simulink model "Flap"  (R2024b)
settings: Solver=ode45  StartTime=0  StopTime=400  FixedStep=0.1  MaxStep=0.1  EnableMultiTasking=on
values from neighbouring files (symbols this model uses):
  Ki = -2*pi/5*imag(1/H(1)')    [BranchAndBound.m]    (also in Optimization.m; RectangularOptimization.m; RoundingPI.m; wecSimInputFile.m = -100000)
  Kp = real(1/H(1)')    [BranchAndBound.m]    (also in Optimization.m; RectangularOptimization.m; RoundingPI.m; wecSimInputFile.m = 500000)
  params = struct    [BranchAndBound.m]    (also in Optimization.m; Parameters.m = struct(); RectangularOptimization.m; RoundingPI.m)
  PTO = 'Continuous PI'    [wecSimInputFile.m]
  valveTransferFunction = tf(4/valveSettlingTime,[1 4/valveSettlingTime])    [Parameters.m]
undefined symbols (not defined in the file or in its folder): body, constraint, geometry, hydroData, pressure, pto, ptoSim
libraries: WECSim_Lib_Body_Elements x2, WECSim_Lib_Constraints x1, WECSim_Lib_Frames x1, simulink x1, WECSim_Lib_PTOSim x1, WECSim_Lib_PTOs x1
(part 2 of 2)

== system Flap/PTO/Active Valving/capValves/Subsystem1 ==
  Pin : Inport
  Pout : Inport  Port=2
  valveCommand : Inport  Port=3
  MATLAB Function : MATLAB Function  TreatAsAtomicUnit=on
  flow : Outport
  loss : Outport  Port=2
  wires:
  MATLAB Function/1(flow) -> flow/1
  valveCommand/1 -> MATLAB Function/3(valveCommand)
  Pout/1 -> MATLAB Function/2(Pout)
  Pin/1 -> MATLAB Function/1(Pin)
  MATLAB Function/2(loss) -> loss/1

== system Flap/PTO/Active Valving/capValves/Subsystem2 ==
  Pin : Inport
  Pout : Inport  Port=2
  valveCommand : Inport  Port=3
  MATLAB Function : MATLAB Function  TreatAsAtomicUnit=on
  flow : Outport
  loss : Outport  Port=2
  wires:
  MATLAB Function/1(flow) -> flow/1
  valveCommand/1 -> MATLAB Function/3(valveCommand)
  Pout/1 -> MATLAB Function/2(Pout)
  Pin/1 -> MATLAB Function/1(Pin)
  MATLAB Function/2(loss) -> loss/1

== system Flap/PTO/Active Valving/rodValves/Subsystem ==
  Pin : Inport
  Pout : Inport  Port=2
  valveCommand : Inport  Port=3
  MATLAB Function : MATLAB Function  TreatAsAtomicUnit=on
  flow : Outport
  loss : Outport  Port=2
  wires:
  MATLAB Function/1(flow) -> flow/1
  valveCommand/1 -> MATLAB Function/3(valveCommand)
  Pout/1 -> MATLAB Function/2(Pout)
  Pin/1 -> MATLAB Function/1(Pin)
  MATLAB Function/2(loss) -> loss/1

== system Flap/PTO/Active Valving/rodValves/Subsystem1 ==
  Pin : Inport
  Pout : Inport  Port=2
  valveCommand : Inport  Port=3
  MATLAB Function : MATLAB Function  TreatAsAtomicUnit=on
  flow : Outport
  loss : Outport  Port=2
  wires:
  MATLAB Function/1(flow) -> flow/1
  valveCommand/1 -> MATLAB Function/3(valveCommand)
  Pout/1 -> MATLAB Function/2(Pout)
  Pin/1 -> MATLAB Function/1(Pin)
  MATLAB Function/2(loss) -> loss/1

== system Flap/PTO/Active Valving/rodValves/Subsystem2 ==
  Pin : Inport
  Pout : Inport  Port=2
  valveCommand : Inport  Port=3
  MATLAB Function : MATLAB Function  TreatAsAtomicUnit=on
  flow : Outport
  loss : Outport  Port=2
  wires:
  MATLAB Function/1(flow) -> flow/1
  valveCommand/1 -> MATLAB Function/3(valveCommand)
  Pout/1 -> MATLAB Function/2(Pout)
  Pin/1 -> MATLAB Function/1(Pin)
  MATLAB Function/2(loss) -> loss/1

== system Flap/PTO/EHA/Subsystem/CapPressureDynamics ==
  position : Inport
  velocity : Inport  Port=2
  flow : Inport  Port=3
  Gain : Gain  Gain=params.capArea
  Integrator : Integrator  LimitOutput=on  UpperSaturationLimit=30e6  LowerSaturationLimit=0
  MATLAB Function : MATLAB Function  TreatAsAtomicUnit=on
  Scope : Scope  NumInputPorts=3
  Subtract : Sum  Inputs=+-
  capPressure : Outport
  wires:
  MATLAB Function/1(pressure_dot) -> Integrator/1
  Integrator/1 -> capPressure/1  "capPressure"
  flow/1 -> Scope/2, Subtract/1, MATLAB Function/3(flow)
  velocity/1 -> Gain/1, MATLAB Function/2(velocity)
  position/1 -> MATLAB Function/1(position)
  Gain/1 -> Subtract/2, Scope/1  "capdV"
  Subtract/1 -> Scope/3  "capQ_dV"

== system Flap/PTO/EHA/Subsystem/HECM ==
  note: dP = capPressure - rodPressure
  displacementCommand : Inport
  rodPressure : Inport  Port=2
  capPressure : Inport  Port=3
  Gain : Gain  Gain=-1
  MATLAB Function : MATLAB Function  TreatAsAtomicUnit=on
  Subtract : Sum  Inputs=+-
  Terminator : Terminator
  Terminator1 : Terminator
  To Workspace : ToWorkspace  VariableName=electricPower  SampleTime=-1
  capFlow : Outport
  rodFlow : Outport  Port=2
  wires:
  Subtract/1 -> MATLAB Function/2(dp)  "dP_actual"
  MATLAB Function/1(Loss) -> Terminator/1  "Loss"
  rodPressure/1 -> Subtract/2
  displacementCommand/1 -> MATLAB Function/1(x)
  MATLAB Function/2(Q) -> rodFlow/1, Gain/1  "rodFlow"
  capPressure/1 -> Subtract/1
  Gain/1 -> capFlow/1  "capFlow"
  MATLAB Function/3(elecPower) -> To Workspace/1, Terminator1/1  "electricPower"

== system Flap/PTO/EHA/Subsystem/RodPressureDynamics ==
  velocity : Inport
  position : Inport  Port=2
  flow : Inport  Port=3
  Integrator : Integrator  LimitOutput=on  UpperSaturationLimit=30e6  LowerSaturationLimit=0
  MATLAB Function : MATLAB Function  TreatAsAtomicUnit=on
  rodPressure : Outport
  wires:
  position/1 -> MATLAB Function/1(position)
  velocity/1 -> MATLAB Function/2(velocity)
  flow/1 -> MATLAB Function/3(flow)
  Integrator/1 -> rodPressure/1  "rodPressure"
  MATLAB Function/1(pressure_dot) -> Integrator/1  "rodPressureDot"

== system Flap/PTO/HHEA/Subsystem/CapPressureDynamics ==
  position : Inport
  velocity : Inport  Port=2
  flow : Inport  Port=3
  Integrator : Integrator
  MATLAB Function : MATLAB Function  TreatAsAtomicUnit=on
  capPressure : Outport
  wires:
  MATLAB Function/1(pressure_dot) -> Integrator/1
  Integrator/1 -> capPressure/1  "capPressure"
  flow/1 -> MATLAB Function/3(flow)
  velocity/1 -> MATLAB Function/2(velocity)
  position/1 -> MATLAB Function/1(position)

== system Flap/PTO/HHEA/Subsystem/HECM ==
  note: dP = rodValvePressure - rodPressure
      | (+) positive dP and torque causes positive flow and speed, which causes increased pressure in the rod chamber
  flowIn : Inport
  speedCommand : Inport  Port=2
  rodPressure : Inport  Port=3
  Integrator : Integrator
  MATLAB Function : MATLAB Function  TreatAsAtomicUnit=on
  MATLAB Function1 : MATLAB Function  TreatAsAtomicUnit=on
  Scope : Scope  NumInputPorts=2
  Scope1 : Scope  NumInputPorts=2
  Subtract : Sum  Inputs=+-
  Terminator : Terminator
  flowOut : Outport
  rodValvePressure : Outport  Port=2
  wires:
  Subtract/1 -> Scope/1, MATLAB Function/2(dp)  "dP_actual"
  MATLAB Function/1(Loss) -> Terminator/1
  MATLAB Function/3(dp_ideal) -> Scope/2
  MATLAB Function/4(w_ideal) -> Scope1/2
  rodPressure/1 -> Subtract/2
  speedCommand/1 -> Scope1/1, MATLAB Function/1(w)
  MATLAB Function/2(Q) -> MATLAB Function1/2(Q_out), flowOut/1  "rodFlow"
  MATLAB Function1/1(Pdot) -> Integrator/1
  Integrator/1 -> Subtract/1, rodValvePressure/1  "rodValvePressure"
  flowIn/1 -> MATLAB Function1/1(Q_in)

== system Flap/PTO/HHEA/Subsystem/PressureRails ==
  note: flow into the rails
  capRailFlow : Inport
  rodRailFlow : Inport  Port=2
  Constant : Constant  Value=35e6
  Constant3 : Constant  Value=17.5e6
  Constant4 : Constant  Value=0
  Mux : Mux  Inputs=3
  Product : Product
  Sum : Sum  Inputs=|++
  Sum of Elements : Sum  Inputs=+
  To Workspace : ToWorkspace  VariableName=railPower  SampleTime=-1
  pressureRails : Outport
  wires:
  Sum/1 -> Product/1
  Product/1 -> Sum of Elements/1
  Sum of Elements/1 -> To Workspace/1
  rodRailFlow/1 -> Sum/2
  capRailFlow/1 -> Sum/1
  Constant3/1 -> Mux/2
  Constant4/1 -> Mux/1
  Constant/1 -> Mux/3
  Mux/1 -> Product/2, pressureRails/1

== system Flap/PTO/HHEA/Subsystem/RodPressureDynamics ==
  velocity : Inport
  position : Inport  Port=2
  flow : Inport  Port=3
  Gain : Gain  Gain=-params.rodArea
  Integrator : Integrator
  MATLAB Function : MATLAB Function  TreatAsAtomicUnit=on
  Scope : Scope  NumInputPorts=2
  Scope1 : Scope  NumInputPorts=2
  Scope2 : Scope
  Sum : Sum  Inputs=|++
  rodPressure : Outport
  wires:
  position/1 -> MATLAB Function/1(position)
  velocity/1 -> MATLAB Function/2(velocity), Gain/1
  flow/1 -> Sum/2, Scope1/2, MATLAB Function/3(flow)
  Integrator/1 -> Scope/2, rodPressure/1  "rodPressure"
  MATLAB Function/1(pressure_dot) -> Scope/1, Integrator/1  "rodPressureDot"
  Gain/1 -> Sum/1, Scope1/1
  Sum/1 -> Scope2/1

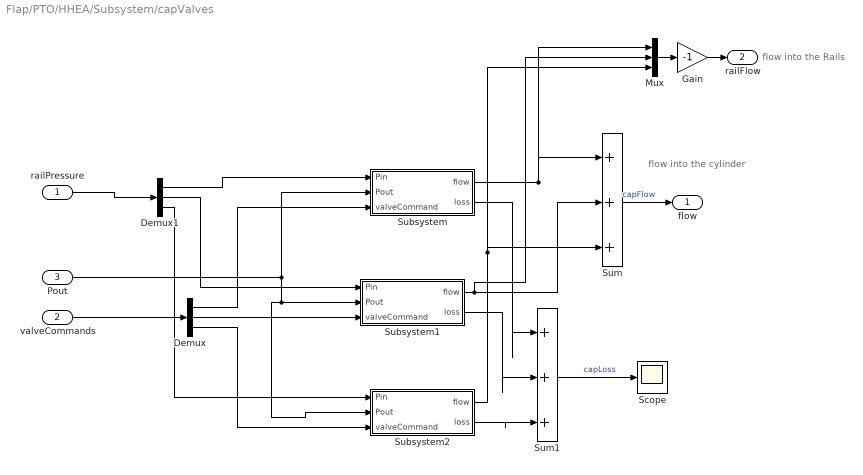
== system Flap/PTO/HHEA/Subsystem/capValves ==
  note: flow into the cylinder
  note: flow into the Rails
  railPressure : Inport
  valveCommands : Inport  Port=2
  Pout : Inport  Port=3
  Demux : Demux  Outputs=3
  Demux1 : Demux  Outputs=3
  Gain : Gain  Gain=-1
  Mux : Mux  Inputs=3
  Scope : Scope
  Subsystem : Subsystem
  Subsystem1 : Subsystem
  Subsystem2 : Subsystem
  Sum : Sum  Inputs=|+++
  Sum1 : Sum  Inputs=|+++
  flow : Outport
  railFlow : Outport  Port=2
  wires:
  Pout/1 -> Subsystem/2(Pout), Subsystem2/2(Pout), Subsystem1/2(Pout)
  valveCommands/1 -> Demux/1
  Demux/1 -> Subsystem/3(valveCommand)
  Demux/2 -> Subsystem1/3(valveCommand)
  Demux/3 -> Subsystem2/3(valveCommand)
  Sum/1 -> flow/1  "capFlow"
  Subsystem/2(loss) -> Sum1/1
  Subsystem1/2(loss) -> Sum1/2
  Subsystem2/2(loss) -> Sum1/3
  Sum1/1 -> Scope/1  "capLoss"
  railPressure/1 -> Demux1/1
  Demux1/1 -> Subsystem/1(Pin)
  Demux1/2 -> Subsystem1/1(Pin)
  Demux1/3 -> Subsystem2/1(Pin)
  Subsystem1/1(flow) -> Mux/2, Sum/2
  Mux/1 -> Gain/1
  Subsystem2/1(flow) -> Mux/3, Sum/3
  Subsystem/1(flow) -> Mux/1, Sum/1
  Gain/1 -> railFlow/1

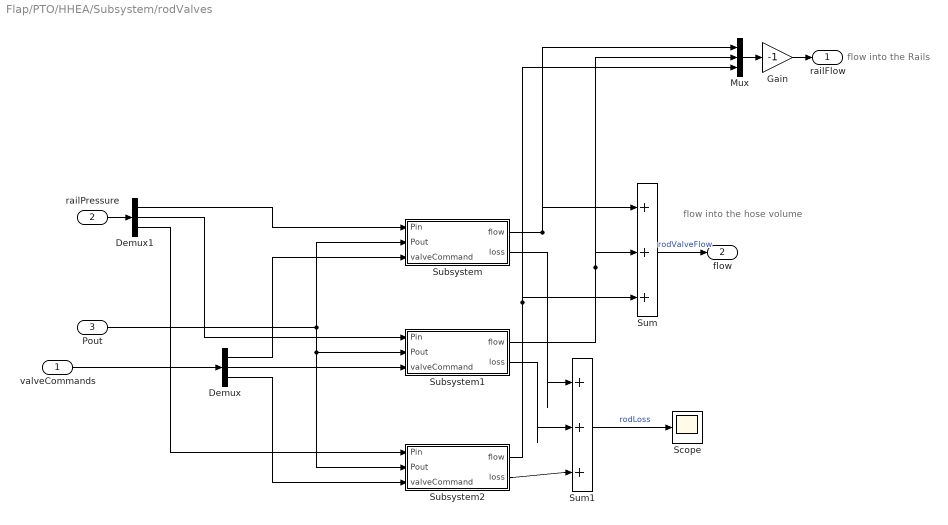
== system Flap/PTO/HHEA/Subsystem/rodValves ==
  note: flow into the hose volume
  note: flow into the Rails
  valveCommands : Inport
  railPressure : Inport  Port=2
  Pout : Inport  Port=3
  Demux : Demux  Outputs=3
  Demux1 : Demux  Outputs=3
  Gain : Gain  Gain=-1
  Mux : Mux  Inputs=3
  Scope : Scope
  Subsystem : Subsystem
  Subsystem1 : Subsystem
  Subsystem2 : Subsystem
  Sum : Sum  Inputs=|+++
  Sum1 : Sum  Inputs=|+++
  railFlow : Outport
  flow : Outport  Port=2
  wires:
  Pout/1 -> Subsystem/2(Pout), Subsystem2/2(Pout), Subsystem1/2(Pout)
  valveCommands/1 -> Demux/1
  Demux/1 -> Subsystem/3(valveCommand)
  Demux1/2 -> Subsystem1/1(Pin)
  Demux1/3 -> Subsystem2/1(Pin)
  Demux/2 -> Subsystem1/3(valveCommand)
  Demux/3 -> Subsystem2/3(valveCommand)
  Sum/1 -> flow/1  "rodValveFlow"
  Subsystem/2(loss) -> Sum1/1
  Subsystem1/2(loss) -> Sum1/2
  Subsystem2/2(loss) -> Sum1/3
  Sum1/1 -> Scope/1  "rodLoss"
  railPressure/1 -> Demux1/1
  Demux1/1 -> Subsystem/1(Pin)
  Subsystem1/1(flow) -> Mux/2, Sum/2
  Mux/1 -> Gain/1
  Subsystem2/1(flow) -> Mux/3, Sum/3
  Subsystem/1(flow) -> Mux/1, Sum/1
  Gain/1 -> railFlow/1

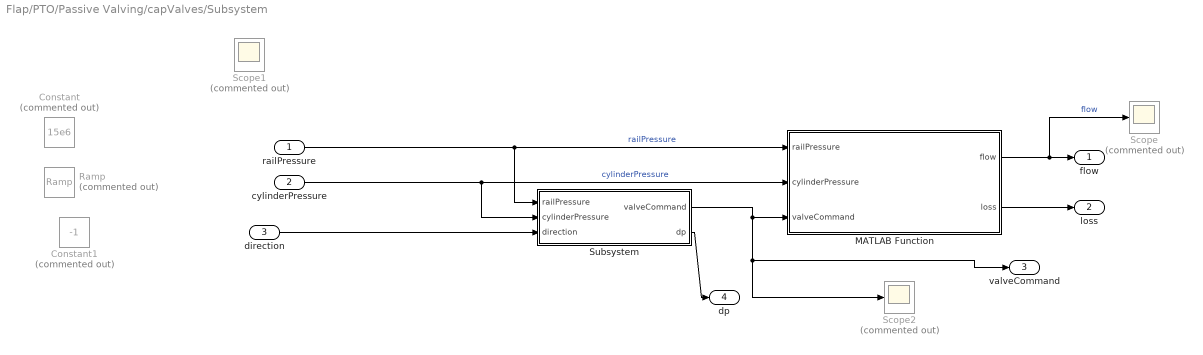
== system Flap/PTO/Passive Valving/capValves/Subsystem ==
  railPressure : Inport
  cylinderPressure : Inport  Port=2
  direction : Inport  Port=3
  Constant : Constant  Commented=on  Value=15e6
  Constant1 : Constant  Commented=on  Value=-1
  MATLAB Function : MATLAB Function  TreatAsAtomicUnit=on
  Ramp : simulink/Sources/Ramp  Commented=on  slope=-1e6  start=0  InitialOutput=20e6
  Scope : Scope  Commented=on
  Scope1 : Scope  Commented=on  NumInputPorts=2
  Scope2 : Scope  Commented=on
  Subsystem : Subsystem
  flow : Outport
  loss : Outport  Port=2
  valveCommand : Outport  Port=3
  dp : Outport  Port=4
  wires:
  railPressure/1 -> Subsystem/1(railPressure), MATLAB Function/1(railPressure)  "railPressure"
  Subsystem/1(valveCommand) -> valveCommand/1, Scope2/1, MATLAB Function/3(valveCommand)
  MATLAB Function/1(flow) -> Scope/1, flow/1  "flow"
  Subsystem/2(dp) -> dp/1
  MATLAB Function/2(loss) -> loss/1
  direction/1 -> Subsystem/3(direction)
  cylinderPressure/1 -> MATLAB Function/2(cylinderPressure), Subsystem/2(cylinderPressure)  "cylinderPressure"

== system Flap/PTO/HHEA/Subsystem/capValves/Subsystem ==
  Pin : Inport
  Pout : Inport  Port=2
  valveCommand : Inport  Port=3
  MATLAB Function : MATLAB Function  TreatAsAtomicUnit=on
  Transfer Fcn : TransferFcn  Numerator=valveTransferFunction.Numerator{1}  Denominator=valveTransferFunction.Denominator{1}
  flow : Outport
  loss : Outport  Port=2
  wires:
  MATLAB Function/1(flow) -> flow/1
  valveCommand/1 -> Transfer Fcn/1
  Pout/1 -> MATLAB Function/2(Pout)
  Pin/1 -> MATLAB Function/1(Pin)
  MATLAB Function/2(loss) -> loss/1
  Transfer Fcn/1 -> MATLAB Function/3(valveCommand)

== system Flap/PTO/HHEA/Subsystem/capValves/Subsystem1 ==
  Pin : Inport
  Pout : Inport  Port=2
  valveCommand : Inport  Port=3
  MATLAB Function : MATLAB Function  TreatAsAtomicUnit=on
  Transfer Fcn : TransferFcn  Numerator=valveTransferFunction.Numerator{1}  Denominator=valveTransferFunction.Denominator{1}
  flow : Outport
  loss : Outport  Port=2
  wires:
  MATLAB Function/1(flow) -> flow/1
  valveCommand/1 -> Transfer Fcn/1
  Pout/1 -> MATLAB Function/2(Pout)
  Pin/1 -> MATLAB Function/1(Pin)
  MATLAB Function/2(loss) -> loss/1
  Transfer Fcn/1 -> MATLAB Function/3(valveCommand)

== system Flap/PTO/HHEA/Subsystem/capValves/Subsystem2 ==
  Pin : Inport
  Pout : Inport  Port=2
  valveCommand : Inport  Port=3
  MATLAB Function : MATLAB Function  TreatAsAtomicUnit=on
  Transfer Fcn : TransferFcn  Numerator=valveTransferFunction.Numerator{1}  Denominator=valveTransferFunction.Denominator{1}
  flow : Outport
  loss : Outport  Port=2
  wires:
  MATLAB Function/1(flow) -> flow/1
  valveCommand/1 -> Transfer Fcn/1
  Pout/1 -> MATLAB Function/2(Pout)
  Pin/1 -> MATLAB Function/1(Pin)
  MATLAB Function/2(loss) -> loss/1
  Transfer Fcn/1 -> MATLAB Function/3(valveCommand)

== system Flap/PTO/HHEA/Subsystem/rodValves/Subsystem ==
  Pin : Inport
  Pout : Inport  Port=2
  valveCommand : Inport  Port=3
  MATLAB Function : MATLAB Function  TreatAsAtomicUnit=on
  Transfer Fcn : TransferFcn  Numerator=valveTransferFunction.Numerator{1}  Denominator=valveTransferFunction.Denominator{1}
  flow : Outport
  loss : Outport  Port=2
  wires:
  MATLAB Function/1(flow) -> flow/1
  valveCommand/1 -> Transfer Fcn/1
  Pout/1 -> MATLAB Function/2(Pout)
  Pin/1 -> MATLAB Function/1(Pin)
  MATLAB Function/2(loss) -> loss/1
  Transfer Fcn/1 -> MATLAB Function/3(valveCommand)

== system Flap/PTO/HHEA/Subsystem/rodValves/Subsystem1 ==
  Pin : Inport
  Pout : Inport  Port=2
  valveCommand : Inport  Port=3
  MATLAB Function : MATLAB Function  TreatAsAtomicUnit=on
  Transfer Fcn : TransferFcn  Numerator=valveTransferFunction.Numerator{1}  Denominator=valveTransferFunction.Denominator{1}
  flow : Outport
  loss : Outport  Port=2
  wires:
  MATLAB Function/1(flow) -> flow/1
  valveCommand/1 -> Transfer Fcn/1
  Pout/1 -> MATLAB Function/2(Pout)
  Pin/1 -> MATLAB Function/1(Pin)
  MATLAB Function/2(loss) -> loss/1
  Transfer Fcn/1 -> MATLAB Function/3(valveCommand)

== system Flap/PTO/HHEA/Subsystem/rodValves/Subsystem2 ==
  Pin : Inport
  Pout : Inport  Port=2
  valveCommand : Inport  Port=3
  MATLAB Function : MATLAB Function  TreatAsAtomicUnit=on
  Transfer Fcn : TransferFcn  Numerator=valveTransferFunction.Numerator{1}  Denominator=valveTransferFunction.Denominator{1}
  flow : Outport
  loss : Outport  Port=2
  wires:
  MATLAB Function/1(flow) -> flow/1
  valveCommand/1 -> Transfer Fcn/1
  Pout/1 -> MATLAB Function/2(Pout)
  Pin/1 -> MATLAB Function/1(Pin)
  MATLAB Function/2(loss) -> loss/1
  Transfer Fcn/1 -> MATLAB Function/3(valveCommand)

== system Flap/PTO/Passive Valving/capValves/Subsystem/Subsystem ==
  note: dp = inlet - outlet
      | Positive dp tends to open the valve and cause flow from the inlet to the outlet
  railPressure : Inport
  cylinderPressure : Inport  Port=2
  direction : Inport  Port=3
  Gain : Gain  Gain=1/params.checkValveStroke
  "Integrator, Second-Order Limited" : SecondOrderIntegrator  LimitX=on  UpperLimitX=params.checkValveStroke  LowerLimitX=0  LimitDXDT=on
  MATLAB Function : MATLAB Function  TreatAsAtomicUnit=on
  MATLAB Function1 : MATLAB Function  TreatAsAtomicUnit=on
  Subtract : Sum  Inputs=+-
  valveCommand : Outport
  dp : Outport  Port=2
  wires:
  "Integrator, Second-Order Limited"/1 -> MATLAB Function/2(x), Gain/1
  "Integrator, Second-Order Limited"/2 -> MATLAB Function/3(v)
  MATLAB Function/1(a) -> "Integrator, Second-Order Limited"/1
  MATLAB Function1/2(Pout) -> Subtract/2
  Subtract/1 -> dp/1, MATLAB Function/1(dp)
  railPressure/1 -> MATLAB Function1/1(railPressure)
  MATLAB Function1/1(Pin) -> Subtract/1
  cylinderPressure/1 -> MATLAB Function1/2(cylinderPressure)
  direction/1 -> MATLAB Function1/3(direction)
  Gain/1 -> valveCommand/1

== matlab function Flap/PTO/Active Valving/capValves/Subsystem2/MATLAB Function ==
  data: Pin input; flow output; Pout input; valveCommand input; params parameter; loss output
function [flow,loss] = fcn(Pin,Pout,valveCommand,params)
dP = Pin-Pout;
flow = valveCommand*params.valveConstant*sqrt(abs(dP))*sign(dP);
loss = (dP)*flow;

== matlab function Flap/PTO/Active Valving/rodValves/Subsystem/MATLAB Function ==
  data: Pin input; flow output; Pout input; valveCommand input; params parameter; loss output
function [flow,loss] = fcn(Pin,Pout,valveCommand,params)
dP = Pin-Pout;
flow = valveCommand*params.valveConstant*sqrt(abs(dP))*sign(dP);
loss = (dP)*flow;

== matlab function Flap/PTO/Active Valving/rodValves/Subsystem1/MATLAB Function ==
  data: Pin input; flow output; Pout input; valveCommand input; params parameter; loss output
function [flow,loss] = fcn(Pin,Pout,valveCommand,params)
dP = Pin-Pout;
flow = valveCommand*params.valveConstant*sqrt(abs(dP))*sign(dP);
loss = (dP)*flow;

== matlab function Flap/PTO/Active Valving/rodValves/Subsystem2/MATLAB Function ==
  data: Pin input; flow output; Pout input; valveCommand input; params parameter; loss output
function [flow,loss] = fcn(Pin,Pout,valveCommand,params)
dP = Pin-Pout;
flow = valveCommand*params.valveConstant*sqrt(abs(dP))*sign(dP);
loss = (dP)*flow;

== matlab function Flap/PTO/Discrete PI/MATLAB Function ==
  data: forceContinuous input; forceDiscrete output; params parameter
function forceDiscrete = fcn(forceContinuous,params)

pressureRails = [0 17.5 35]*1e6; % [Pa]
capForce = params.capArea *pressureRails;
rodForce = params.rodArea *pressureRails;

forceOptionsMatrix = capForce - rodForce';
forceOptionsVector = forceOptionsMatrix(:);

[~,ind] = min(abs(forceOptionsVector - forceContinuous));
forceDiscrete = forceOptionsVector(ind);

== matlab function Flap/PTO/EHA/Subsystem/CapPressureDynamics/MATLAB Function ==
  data: position input; velocity input; pressure_dot output; flow input; params parameter
function pressure_dot = CapPressure(position,velocity,flow,params)
% This code calculates the pressure dynamics on the cap side of the cylinder
% flow is flow into the cap side from the valves
% rod side is connected to the flap, positive velocity is extension

%Position is measured from mid stroke. Positive is in extention

volume = params.rodArea*(params.cylinderStroke/2 + position);
pressure_dot = params.beta/volume * (flow - velocity*params.rodArea);

== matlab function Flap/PTO/EHA/Subsystem/HECM/MATLAB Function ==
  data: Loss output; Q output; x input; dp input; params parameter; elecPower output
function [Loss,Q,elecPower] = fcn(x,dp,params)
% x is fractional displacement => from -1 to 1
    % positive fractional displacement results from the cap to the rod
% dp is pressure difference (cap - rod)

w = params.maxMotorSpeed; % [rad/s]
QIdeal = params.Disp*params.maxMotorSpeed*x;
TIdeal = params.Disp*dp*x;


%% EHA Losses
% Variable Displacement Axial Piston, 107 cc/rev (Pourmovahed et al. 1992b)
    D = 107; % cc/rev
    d = (D*100^-3)/(2*pi); % m^3/rad 
% Torques Loss Constants
    Cf =  53.7e-3;
    Ch = 53.6;
    Cv = 23.5e3;
% Flow Loss Constants
    Cs = 4.26e-9;
    Cst = 0*1e-5;
% Fluid Properties
    mu=(32e-6)*870;
    rho = 870;
% Losses
    QLoss = params.scaleHECM*abs(d*Cs*dp/mu) + params.scaleHECM*abs(x*d*w*dp/params.beta) + params.scaleHECM*abs(d^(2/3)*Cst*(2*abs(dp)/rho)^.5);
    TLoss = params.scaleHECM*(  abs(d*Cv*mu*w) + abs(d*dp*Cf) + abs(x*Ch*w^2*rho*d^(5/3)/2)  );

% Losses added with sign convention of a motor
    % positive x, and dp is motoring.
        % x>0 sends flow from the cap side to the rod side, which if dp>0, means high pressure to low pressure (motoring)
            % |Q| should be more than |QIdeal| and |T| should be less than |TIdeal|
        % x<0 sends flow from the rod side to the cap side, which if dp>0, means low pressure to high pressure (pumping)
            % |Q| should be less than |QIdeal| and |T| should be more than |TIdeal|
    Q = QIdeal + sign(dp)*QLoss;
    T = TIdeal - sign(w)*TLoss;

% Hydraulic Loss
    % if motoring, Q*dp is positve and smaller in magnitude that w*T
    % if pumping, Q*dp is negative and larger in magnitude that w*T
    hydrLoss = abs(w*T - Q*dp); 
    
% Electric Loss
    % Constant 90% effiency
    if w*T > 0 % motoring
        elecPower = .9*w*T; 
        elecLoss = .1*w*T; % Loss incurred going from shaft power to electric power
    else % pumping
        elecPower = w*T/.9; % There is an amount of electric power than when it goes through the 90% eff e-motor, will give w*T shaft power
        elecLoss = (1/.9-1)*(-w*T);
    end

% Total Loss
Loss = hydrLoss + elecLoss;

== matlab function Flap/PTO/EHA/Subsystem/RodPressureDynamics/MATLAB Function ==
  data: position input; velocity input; pressure_dot output; flow input; params parameter
function pressure_dot = RodPressure(position,velocity,flow,params)
% This code calculates the pressure dynamics on the rod side of the cylinder
% flow is flow into the rod side from the valves
% rod side is connected to the flap, positive velocity is extension

% Position is measured from mid stroke. Positive is in extention
volume = params.capArea*( params.cylinderStroke/2 - position);
pressure_dot = params.beta/volume * (flow + velocity*params.rodArea);

== matlab function Flap/PTO/HHEA/Controller/MATLAB Function ==
  data: forceDiscrete output; capValveCommands output; rodValveCommands output; forceContinuous input; pressureRails input; capPressure input; rodValvePressure input; params parameter; rodPressureCommand output
function [forceDiscrete,capValveCommands,rodValveCommands,rodPressureCommand] = fcn(forceContinuous, pressureRails,capPressure,rodValvePressure,params)
%% pressure Rail Commands
% pressureRails = [0; 15; 30]*1e6; % [Pa]
capForce = params.capArea *pressureRails;
rodForce = params.rodArea *pressureRails;

forceOptionsMatrix = capForce' - rodForce;
rodPressureCommand = -1; % initialize
ind = NaN; forceDiscrete = NaN;capValveCommands = zeros(size(pressureRails)); rodValveCommands = zeros(size(pressureRails)); dP_command = NaN;
while rodPressureCommand < 0
[~,ind] = min(abs(forceOptionsMatrix-forceContinuous),[],'all');
[rodInd,capInd] = ind2sub(size(forceOptionsMatrix),ind);
forceDiscrete = params.capArea *pressureRails(capInd) - params.rodArea *pressureRails(rodInd);

% make bus to send to valves
capValveCommands = zeros(size(pressureRails)); capValveCommands(capInd) = 1;
rodValveCommands = zeros(size(pressureRails)); rodValveCommands(rodInd) = 1;

% Hecm command
dP_commandIdeal = (forceContinuous-forceDiscrete) / params.rodArea;
rodPressureCommand = rodValvePressure - dP_commandIdeal;

% assign that entry to NaN for the next loop in case rodPressure is less than zero,
forceOptionsMatrix(ind) = NaN;

if sum(isfinite(forceOptionsMatrix(:))) == 0
    forceContinuous, pressureRails,capPressure,rodValvePressure
    %error('Negative pressure command')
    dP_command = rodValvePressure;
    rodPressureCommand = rodValvePressure - dP_command;
end

end

% check that dP_command gets to the continuous force
[capPressure*params.capArea - rodPressureCommand*params.rodArea, forceContinuous];

% Actual Hecm command
forceDiscreteActual = params.capArea*capPressure - rodValvePressure *params.rodArea;
dP_command = (forceContinuous-forceDiscreteActual) / params.rodArea;

rodPressureCommand = rodValvePressure - dP_command;

== matlab function Flap/PTO/HHEA/Subsystem/CapPressureDynamics/MATLAB Function ==
  data: position input; velocity input; pressure_dot output; flow input; params parameter
function pressure_dot = CapPressure(position,velocity,flow,params)
% This code calculates the pressure dynamics on the cap side of the cylinder
% flow is flow into the cap side from the valves
% rod side is connected to the flap, positive velocity is extension

%Position is measured from mid stroke. Positive is in extention

volume = params.capArea*(params.cylinderStroke/2 + position);
pressure_dot = params.beta/volume * (flow - velocity*params.capArea);

== matlab function Flap/PTO/Passive Valving/capValves/Subsystem/Subsystem/MATLAB Function1 ==
  data: railPressure input; Pin output; cylinderPressure input; direction input; Pout output
function [Pin,Pout] = fcn(railPressure, cylinderPressure, direction)
% positive "direction" allows flow into the cylinder
if direction > 0
    Pin = railPressure;
    Pout = cylinderPressure;
else
    Pin = cylinderPressure;
    Pout = railPressure;
end

== matlab function Flap/PTO/HHEA/Subsystem/HECM/MATLAB Function ==
  data: Loss output; Q output; dp_ideal output; w input; dp input; params parameter; w_ideal output
function [Loss,Q,dp_ideal,w_ideal] = fcn(w,dp,params)
% pump map is loaded in parameters script
% sign convention is that of a pump

Q = params.scaleHECM*interp2(params.P1_Mapping,params.w1rad_Mapping,params.Q1_Act_Mapping,dp,w);
T = params.scaleHECM*interp2(params.P1_Mapping,params.w1rad_Mapping,params.T1_Act_Mapping,dp,w);

Loss = T*w-dp*Q;

% check that it makes sense
dp_ideal = T/params.Disp;
w_ideal = Q/params.Disp;

== matlab function Flap/PTO/HHEA/Subsystem/HECM/MATLAB Function1 ==
  data: Q_in input; Pdot output; Q_out input; params parameter
function Pdot = fcn(Q_in,Q_out,params)

Pdot = params.beta/params.hoseVolume*(Q_in-Q_out);

== matlab function Flap/PTO/HHEA/Subsystem/RodPressureDynamics/MATLAB Function ==
  data: position input; velocity input; pressure_dot output; flow input; params parameter
function pressure_dot = RodPressure(position,velocity,flow,params)
% This code calculates the pressure dynamics on the rod side of the cylinder
% flow is flow into the rod side from the valves
% rod side is connected to the flap, positive velocity is extension

% Position is measured from mid stroke. Positive is in extention
volume = params.capArea*( params.cylinderStroke/2 - position);
pressure_dot = params.beta/volume * (flow + velocity*params.rodArea);

== matlab function Flap/PTO/HHEA/Subsystem/capValves/Subsystem/MATLAB Function ==
  data: Pin input; flow output; Pout input; valveCommand input; params parameter; loss output
function [flow,loss] = fcn(Pin,Pout,valveCommand,params)
dP = Pin-Pout;
flow = valveCommand*params.valveConstant*sqrt(abs(dP))*sign(dP);
loss = (dP)*flow;

== matlab function Flap/PTO/HHEA/Subsystem/capValves/Subsystem1/MATLAB Function ==
  data: Pin input; flow output; Pout input; valveCommand input; params parameter; loss output
function [flow,loss] = fcn(Pin,Pout,valveCommand,params)
dP = Pin-Pout;
flow = valveCommand*params.valveConstant*sqrt(abs(dP))*sign(dP);
loss = (dP)*flow;

== matlab function Flap/PTO/HHEA/Subsystem/capValves/Subsystem2/MATLAB Function ==
  data: Pin input; flow output; Pout input; valveCommand input; params parameter; loss output
function [flow,loss] = fcn(Pin,Pout,valveCommand,params)
dP = Pin-Pout;
flow = valveCommand*params.valveConstant*sqrt(abs(dP))*sign(dP);
loss = (dP)*flow;

== matlab function Flap/PTO/HHEA/Subsystem/rodValves/Subsystem/MATLAB Function ==
  data: Pin input; flow output; Pout input; valveCommand input; params parameter; loss output
function [flow,loss] = fcn(Pin,Pout,valveCommand,params)
dP = Pin-Pout;
flow = valveCommand*params.valveConstant*sqrt(abs(dP))*sign(dP);
loss = (dP)*flow;

== matlab function Flap/PTO/HHEA/Subsystem/rodValves/Subsystem1/MATLAB Function ==
  data: Pin input; flow output; Pout input; valveCommand input; params parameter; loss output
function [flow,loss] = fcn(Pin,Pout,valveCommand,params)
dP = Pin-Pout;
flow = valveCommand*params.valveConstant*sqrt(abs(dP))*sign(dP);
loss = (dP)*flow;

== matlab function Flap/PTO/HHEA/Subsystem/rodValves/Subsystem2/MATLAB Function ==
  data: Pin input; flow output; Pout input; valveCommand input; params parameter; loss output
function [flow,loss] = fcn(Pin,Pout,valveCommand,params)
dP = Pin-Pout;
flow = valveCommand*params.valveConstant*sqrt(abs(dP))*sign(dP);
loss = (dP)*flow;

== matlab function Flap/PTO/Passive Valving/capValves/Subsystem/Subsystem/MATLAB Function ==
  data: dp input; a output; x input; v input; params parameter
function a = fcn(dp,x,v,params)

stroke = params.checkValveStroke;
A = pi*(3*.0254)^2;
m = 7939*A*stroke;
Pc = params.checkValveCrackingPressure;
k = Pc*A/stroke;
c = 2*sqrt(k*m); % critically damped
springPreset = Pc*A ;

a = 1/m * (dp*A -k*x - c*v - springPreset);

== matlab function Flap/PTO/Passive Valving/CapPressureDynamics/MATLAB Function ==
  data: position input; velocity input; pressure_dot output; flow input; params parameter
function pressure_dot = CapPressure(position,velocity,flow,params)
% This code calculates the pressure dynamics on the cap side of the cylinder
% flow is flow into the cap side from the valves
% rod side is connected to the flap, positive velocity is extension

%Position is measured from mid stroke. Positive is in extention

volume = params.capArea*(params.cylinderStroke/2 + position);
pressure_dot = params.beta/volume * (flow - velocity*params.capArea);

== matlab function Flap/PTO/Passive Valving/RodPressureDynamics/MATLAB Function ==
  data: position input; velocity input; pressure_dot output; flow input; params parameter
function pressure_dot = RodPressure(position,velocity,flow,params)
% This code calculates the pressure dynamics on the rod side of the cylinder
% flow is flow into the rod side from the valves
% rod side is connected to the flap, positive velocity is extension

% Position is measured from mid stroke. Positive is in extention
volume = params.capArea*( params.cylinderStroke/2 - position);
pressure_dot = params.beta/volume * (flow + velocity*params.rodArea);

== matlab function Flap/PTO/Rectifying/MATLAB Function ==
  data: velocity input; forceRectified output; params parameter; pressure input
function forceRectified = fcn(velocity,params, pressure)

% positive velocity is extention - give pressure to rod side
forceRectified = -params.rodArea*pressure * (velocity >= 0) + ...
                  params.capArea*pressure * (velocity < 0);

== matlab function Flap/PTO/Passive Valving/capValves/Subsystem/MATLAB Function ==
  data: railPressure input; flow output; cylinderPressure input; valveCommand input; params parameter; loss output
function [flow,loss] = fcn(railPressure,cylinderPressure,valveCommand,params)
dP = railPressure-cylinderPressure;
flow = valveCommand*params.valveConstant*sqrt(abs(dP))*sign(dP);
loss = (dP)*flow;

== matlab function Flap/PTO/Active Valving/CapPressureDynamics/MATLAB Function ==
  data: position input; velocity input; pressure_dot output; flow input; params parameter
function pressure_dot = CapPressure(position,velocity,flow,params)
% This code calculates the pressure dynamics on the cap side of the cylinder
% flow is flow into the cap side from the valves
% rod side is connected to the flap, positive velocity is extension

%Position is measured from mid stroke. Positive is in extention

volume = params.capArea*(params.cylinderStroke/2 + position);
pressure_dot = params.beta/volume * (flow - velocity*params.capArea);

== matlab function Flap/PTO/Active Valving/Controller/MATLAB Function ==
  data: capValveCommands output; rodValveCommands output; forceContinuous input; pressureRails input; forceDiscrete output; params parameter; capPressureCommand output; rodPressureCommand output
function [capValveCommands,rodValveCommands,forceDiscrete,capPressureCommand,rodPressureCommand] = fcn(forceContinuous,pressureRails,params)

% pressureRails = [0; 15; 30]*1e6; % [Pa]
capForce = params.capArea *pressureRails;
rodForce = params.rodArea *pressureRails;

forceOptionsMatrix = capForce' - rodForce;

[~,ind] = min(abs(forceOptionsMatrix-forceContinuous),[],'all');
[rodInd,capInd] = ind2sub(size(forceOptionsMatrix),ind);
forceDiscrete = params.capArea *pressureRails(capInd) - params.rodArea *pressureRails(rodInd);

% make bus to send to valves
capValveCommands = zeros(size(pressureRails)); capValveCommands(capInd) = 1;
rodValveCommands = zeros(size(pressureRails)); rodValveCommands(rodInd) = 1;

capPressureCommand = pressureRails(capInd);
rodPressureCommand = pressureRails(rodInd);

== matlab function Flap/PTO/Active Valving/RodPressureDynamics/MATLAB Function ==
  data: position input; velocity input; pressure_dot output; flow input; params parameter
function pressure_dot = RodPressure(position,velocity,flow,params)
% This code calculates the pressure dynamics on the rod side of the cylinder
% flow is flow into the rod side from the valves
% rod side is connected to the flap, positive velocity is extension

% Position is measured from mid stroke. Positive is in extention
volume = params.capArea*( params.cylinderStroke/2 - position);
pressure_dot = params.beta/volume * (flow + velocity*params.rodArea);

== matlab function Flap/PTO/Active Valving/capValves/Subsystem/MATLAB Function ==
  data: Pin input; flow output; Pout input; valveCommand input; params parameter; loss output
function [flow,loss] = fcn(Pin,Pout,valveCommand,params)
dP = Pin-Pout;
flow = valveCommand*params.valveConstant*sqrt(abs(dP))*sign(dP);
loss = (dP)*flow;

== matlab function Flap/PTO/Active Valving/capValves/Subsystem1/MATLAB Function ==
  data: Pin input; flow output; Pout input; valveCommand input; params parameter; loss output
function [flow,loss] = fcn(Pin,Pout,valveCommand,params)
dP = Pin-Pout;
flow = valveCommand*params.valveConstant*sqrt(abs(dP))*sign(dP);
loss = (dP)*flow;
